simulink model "demo"  (R2016b)
settings: Solver=FixedStepDiscrete  StartTime=0.0  StopTime=10.0  FixedStep=0.01  RelTol=1e-3
values from neighbouring files (symbols this model uses):
  prob = test_problem(N, nx, nu, ny, nc)    [main.m]
undefined symbols (not defined in the file): N, nc, nu, nx, ny, verbose
settings Model: Creator=jgillis  LastModifiedBy=jgillis

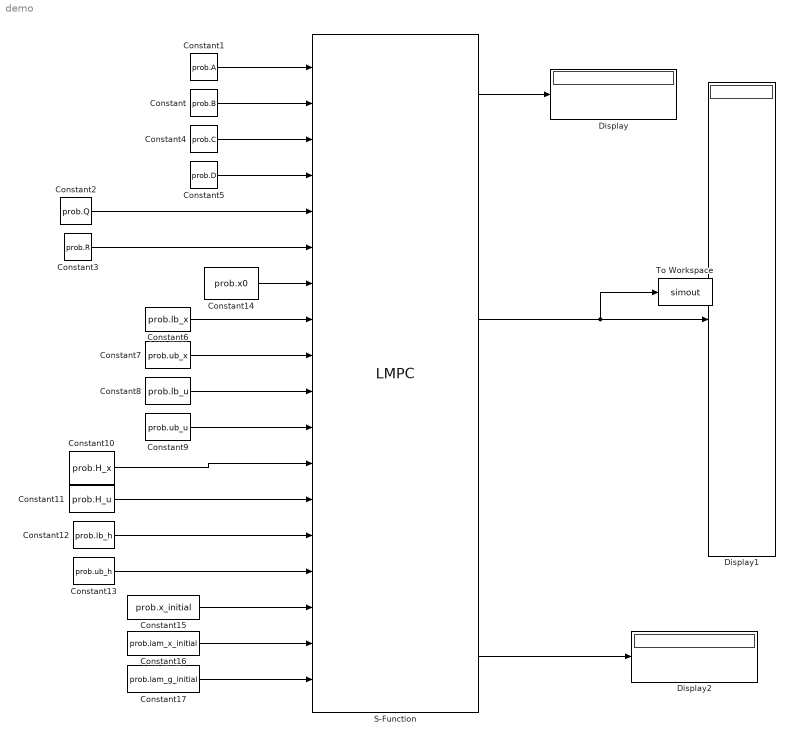
== system demo ==
  Constant : Constant  Value=prob.B
  Constant1 : Constant  Value=prob.A
  Constant10 : Constant  Value=prob.H_x
  Constant11 : Constant  Value=prob.H_u
  Constant12 : Constant  Value=prob.lb_h
  Constant13 : Constant  Value=prob.ub_h
  Constant14 : Constant  Value=prob.x0
  Constant15 : Constant  Value=prob.x_initial
  Constant16 : Constant  Value=prob.lam_x_initial
  Constant17 : Constant  Value=prob.lam_g_initial
  Constant2 : Constant  Value=prob.Q
  Constant3 : Constant  Value=prob.R
  Constant4 : Constant  Value=prob.C
  Constant5 : Constant  Value=prob.D
  Constant6 : Constant  Value=prob.lb_x
  Constant7 : Constant  Value=prob.ub_x
  Constant8 : Constant  Value=prob.lb_u
  Constant9 : Constant  Value=prob.ub_u
  Display : Display
  Display1 : Display
  Display2 : Display
  S-Function : S-Function  FunctionName=LMPC  SFunctionModules='MPC_step'  SFunctionDeploymentMode=off  EnableBusSupport=off  mask{N=N, nx=nx, nu=nu, ny=ny, nc=nc, max_iter=1000, constr_viol_tol=1e-8, dual_inf_tol=1e-8, verbose=verbose}
      mask prompts: N "N (horizon size)"; nx "nx (number of states)"; nu "nu (number of controls)"; ny "ny (number of outputs)"; nc "nc (number of constraints)"
      mask init:
      | f = generate_block(N,nx,nu,ny,nc,max_iter,constr_viol_tol,dual_inf_tol,verbose);
      | 
      | s = '';
      | for i=1:f.n_in
      |    s = [s sprintf('port_label(''input'',%d,''%s %s'');\n',i,f.name_in(i-1),dim(f.sparsity_in(i-1)))];
      | end
      | for i=1:f.n_out
      |    s = [s sprintf('port_label(''output'',%d,''%s %s'');\n',i,f.name_out(i-1),dim(f.sparsity_out(i-1)))];
      | end
      | 
      | s = [s sprintf('port_label(''output'',%d,''%s'');\n',f.n_out+1,'is_fail?')];
      | 
      | set_param(gcb,'maskDisplay',s);
      mask Display:
      | port_label('input',1,'A 5x5');
      | port_label('input',2,'B 5x2');
      | port_label('input',3,'C 1x5');
      | port_label('input',4,'D 1x2');
      | port_label('input',5,'Q 5x5');
      | port_label('input',6,'R 2x2');
      | port_label('input',7,'x0 5x1');
      | port_label('input',8,'lb_x 5x1');
      | port_label('input',9,'ub_x 5x1');
      | port_label('input',10,'lb_u 2x1');
      | port_label('input',11,'ub_u 2x1');
      | port_label('input',12,'H_x 1x5');
      | port_label('input',13,'H_u 1x2');
      | port_label('input',14,'lb_h 1x1');
      | port_label('input',15,'ub_h 1x1');
      | port_label('input',16,'x_initial 40x1');
      | port_label('input',17,'lam_x_initial 40x1');
      | port_label('input',18,'lam_g_initial 30x1');
      | port_label('output',1,'u_next 2x1');
      | port_label('output',2,'f 1x1');
      | port_label('output',3,'x 40x1');
      | port_label('output',4,'lam_x 40x1');
      | port_label('output',5,'lam_g 30x1');
      | port_label('output',6,'is_fail?');
  To Workspace : ToWorkspace  VariableName=simout  SaveFormat=Timeseries  SampleTime=-1
  wires:
  S-Function/6 -> Display2/1
  Constant1/1 -> S-Function/1
  Constant/1 -> S-Function/2
  Constant2/1 -> S-Function/5
  Constant3/1 -> S-Function/6
  Constant4/1 -> S-Function/3
  Constant5/1 -> S-Function/4
  S-Function/1 -> Display/1
  S-Function/3 -> To Workspace/1, Display1/1
  Constant6/1 -> S-Function/8
  Constant7/1 -> S-Function/9
  Constant8/1 -> S-Function/10
  Constant9/1 -> S-Function/11
  Constant10/1 -> S-Function/12
  Constant11/1 -> S-Function/13
  Constant12/1 -> S-Function/14
  Constant13/1 -> S-Function/15
  Constant14/1 -> S-Function/7
  Constant15/1 -> S-Function/16
  Constant17/1 -> S-Function/18
  Constant16/1 -> S-Function/17
